simulink model "sim_p_regler_reale_strecke"  (R2016b)
settings: Solver=VariableStepAuto  StartTime=0.0  StopTime=20  FixedStep=1e-3  RelTol=1e3
undefined symbols (not defined in the file or in its folder): param
libraries: simulink x5, simulink_extras x1
settings Model: Creator=nicol  LastModifiedBy=Fritz

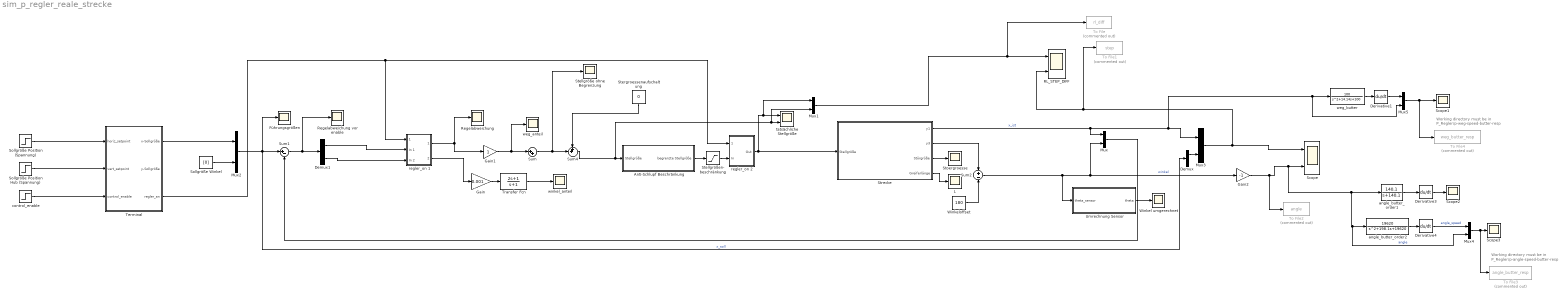
== system sim_p_regler_reale_strecke ==
  note: Working directory must be in
      | P_Regler/p-angle-speed-butter-resp
  note: Working directory must be in
      | P_Regler/p-weg-speed-butter-resp
  Anti-Schlupf Beschränkung : Subsystem
  Demux : Demux  Outputs=2
  Demux1 : Demux  Outputs=2
  Derivative1 : Derivative
  Derivative3 : Derivative
  Derivative4 : Derivative
  Führungsgrößen : Scope
  Gain : Gain  Gain=0.001
  Gain1 : Gain
  Gain2 : Gain  Gain=-1
  L : Scope
  Mux{,1..5} (6 alike) : Mux  Inputs=2
  RL_STEP_DIFF : Scope  NumInputPorts=2
  Regelabweichung : Scope
  Regelabweichung vor enable : Scope
  Scope : Scope  NumInputPorts=2
  Scope1 : Scope
  Scope2 : Scope
  Scope3 : Scope
  Sollgröße Position (Spannung) : Step  SampleTime=0
  Sollgröße Position Hub (Spannung) : Step  Time=2  After=0.5  SampleTime=0
  Sollgröße Winkel : Constant  Value=[0]  VectorParams1D=off
  Stellgröße ohne Begrenzung : Scope
  Stellgrößen- beschränkung : Saturate  UpperLimit=1  LowerLimit=-1
  Stergroessenaufschaltung : Constant  Value=0
  Stoergroesse : Scope
  Strecke : Subsystem
  Sum : Sum  Inputs=|++
  Sum1 : Sum  Inputs=|+-
  Sum2 : Sum  Inputs=+|-
  Sum4 : Sum  Inputs=++|
  Terminal : Subsystem
  To File : ToFile  Commented=on  Filename=rl_diff  SaveFormat=Timeseries
  To File1 : ToFile  Commented=on  Filename=step  SaveFormat=Timeseries
  To File2 : ToFile  Commented=on  Filename=angle  SaveFormat=Timeseries
  To File3 : ToFile  Commented=on  Filename=angle_butter_resp  SaveFormat=Timeseries
  To File4 : ToFile  Commented=on  Filename=weg_butter_resp  SaveFormat=Timeseries
  Transfer Fcn : TransferFcn  Numerator=[2 1]  Denominator=[1 1]
  Umrechnung Sensor : MATLAB Function  TreatAsAtomicUnit=on
  Winkel umgerechnet : Scope
  Winkeloffset : Constant  Value=180
  angle_butter_order1 : TransferFcn  Numerator=[140.1]  Denominator=[1, 140.1]
  angle_butter_order2 : TransferFcn  Numerator=[19620]  Denominator=[1, 198.1, 19620]
  control_enable : Step  Time=0  SampleTime=0
  regler_on 1 : Subsystem
  regler_on 2 : Subsystem
  tatsächliche Stellgröße : Scope  NumInputPorts=2
  weg_anteil : Scope
  weg_butter : TransferFcn  Numerator=[100]  Denominator=[1, 14.14, 100]
  winkel_anteil : Scope
  wires:
  Sum/1 -> Stellgröße ohne Begrenzung/1, Sum4/2
  Sollgröße Winkel/1 -> Mux2/2
  Umrechnung Sensor/1(theta) -> Winkel umgerechnet/1
  Winkeloffset/1 -> Sum2/2
  Sum2/1 -> Umrechnung Sensor/1(theta_sensor), Mux/2, Gain2/1  "winkel"
  Anti-Schlupf Beschränkung/1(begrenzte Stellgröße) -> Stellgrößen- beschränkung/1
  Demux1/1 -> regler_on 1/2(In 1)
  Demux1/2 -> regler_on 1/3(In 2)
  Sum1/1 -> Demux1/1, Regelabweichung vor enable/1
  Mux2/1 -> Demux/1, Sum1/1, Führungsgrößen/1  "x_soll"
  Strecke/1(y1) -> Mux/1, Mux5/2, weg_butter/1, Mux3/1  "x_ist"
  Terminal/3(regler_an) -> regler_on 1/1(regler_ on), regler_on 2/1(regler_ on)
  Strecke/2(y3) -> Sum2/1
  regler_on 1/2(Out 2) -> Gain/1
  regler_on 1/1(Out 1) -> Gain1/1, Regelabweichung/1
  Stellgrößen- beschränkung/1 -> regler_on 2/2(In)
  Sollgröße Position (Spannung)/1 -> Terminal/1(horiz_setpoint)
  control_enable/1 -> Terminal/3(control_enable)
  Sollgröße Position Hub (Spannung)/1 -> Terminal/2(vert_setpoint)
  Terminal/1(x-Sollgröße) -> Mux2/1
  Stergroessenaufschaltung/1 -> Sum4/1
  Strecke/3(Störgröße) -> Stoergroesse/1
  Strecke/4(Greiferlänge) -> L/1
  Mux/1 -> Sum1/2
  Gain/1 -> Transfer Fcn/1
  regler_on 2/1(Out) -> Strecke/1(Stellgröße), Mux1/1, tatsächliche Stellgröße/1
  Sum4/1 -> Mux1/2, tatsächliche Stellgröße/2, Anti-Schlupf Beschränkung/1(Stellgröße)
  Gain1/1 -> weg_anteil/1, Sum/1
  Demux/1 -> Mux3/2
  Mux3/1 -> To File1/1, RL_STEP_DIFF/2, Scope/1
  Mux1/1 -> To File/1, RL_STEP_DIFF/1
  Transfer Fcn/1 -> winkel_anteil/1
  angle_butter_order1/1 -> Derivative3/1
  Derivative3/1 -> Scope2/1
  angle_butter_order2/1 -> Derivative4/1
  Derivative4/1 -> Mux4/1  "angle_speed"
  Gain2/1 -> To File2/1, Mux4/2, angle_butter_order2/1, angle_butter_order1/1, Scope/2  "angle"
  Mux4/1 -> To File3/1, Scope3/1
  weg_butter/1 -> Derivative1/1
  Derivative1/1 -> Mux5/1
  Mux5/1 -> To File4/1, Scope1/1

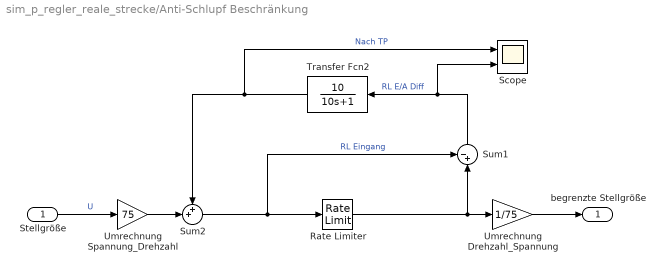
== system sim_p_regler_reale_strecke/Anti-Schlupf Beschränkung ==
  Stellgröße : Inport
  Rate Limiter : RateLimiter  RisingSlewLimit=9.57  FallingSlewLimit=-9.57  SampleTimeMode=inherited
  Scope : Scope  NumInputPorts=2
  Sum1 : Sum  Inputs=-+|
  Sum2 : Sum  Inputs=++|
  Transfer Fcn2 : TransferFcn  Numerator=[10]  Denominator=[10 1]
  Umrechnung Drehzahl_Spannung : Gain  Gain=1/75
  Umrechnung Spannung_Drehzahl : Gain  Gain=75
  begrenzte Stellgröße : Outport
  wires:
  Stellgröße/1 -> Umrechnung Spannung_Drehzahl/1  "U"
  Sum2/1 -> Sum1/1, Rate Limiter/1  "RL Eingang"
  Sum1/1 -> Scope/2, Transfer Fcn2/1  "RL E/A Diff"
  Transfer Fcn2/1 -> Scope/1, Sum2/1  "Nach TP"
  Rate Limiter/1 -> Umrechnung Drehzahl_Spannung/1, Sum1/2
  Umrechnung Spannung_Drehzahl/1 -> Sum2/2
  Umrechnung Drehzahl_Spannung/1 -> begrenzte Stellgröße/1

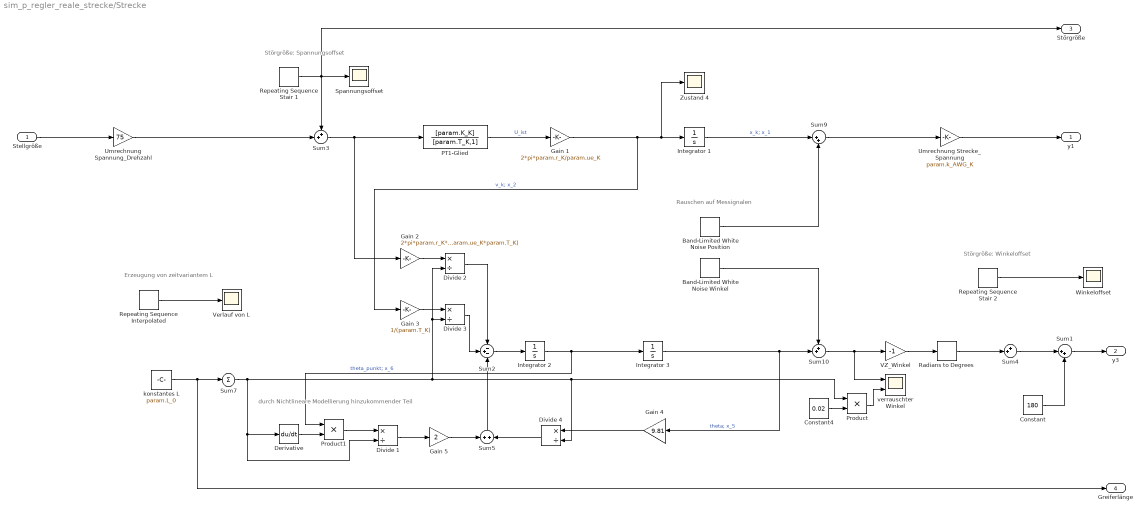
== system sim_p_regler_reale_strecke/Strecke ==
  note: Störgröße: Spannungsoffset
  note: durch Nichtlineare Modellierung hinzukommender Teil
  note: Rauschen auf Messignalen
  note: Erzeugung von zeitvariantem L
  note: Störgröße: Winkeloffset
  Stellgröße : Inport
  Band-Limited White Noise Position : simulink/Sources/Band-Limited White Noise  Cov=[0.0000001]  Ts=0.01  seed=[23341]
  Band-Limited White Noise Winkel : simulink/Sources/Band-Limited White Noise  Cov=[0.000000001]  Ts=0.01  seed=[23341]
  Constant : Constant  Value=180
  Constant4 : Constant  Value=0.02
  Derivative : Derivative
  Divide {1..4} (4 alike) : Product  Inputs=*/
  Gain 1 : Gain  Gain=2*pi*param.r_K/param.ue_K
  Gain 2 : Gain  Gain=2*pi*param.r_K*param.K_K/(param.ue_K*param.T_K)
  Gain 3 : Gain  Gain=1/(param.T_K)
  Gain 4 : Gain  Gain=9.81
  Gain 5 : Gain  Gain=2
  Integrator 1 : Integrator
  Integrator 2 : Integrator
  Integrator 3 : Integrator
  PT1-Glied : TransferFcn  Numerator=[param.K_K]  Denominator=[param.T_K,1]
  Product : Product
  Product1 : Product
  Radians to Degrees : simulink_extras/Transformations/Radians to Degrees
  Repeating Sequence Interpolated : simulink/Sources/Repeating Sequence Interpolated  OutValues=[1.5 1.0 0.7 0.5 0.4 0.3 0.2 0.5 1.5 1.0 0.2 0.2 1.0 1.5 0.5 0.2].'  TimeValues=[0 2 4 6 8 10 12 14 16 18 20 22 24 26 28 30].'  LookUpMeth=Interpolation-Use End Values  tsamp=0.001  OutMin=[]  OutMax=[]  OutDataTypeStr=double  OutputDataTypeScalingMode=double  OutDataType=fixdt(0,8)  OutScaling=2^-10
  Repeating Sequence Stair 1 : simulink/Sources/Repeating Sequence Stair  OutValues=[0.05 0.05 0.05 0.05 0.05].'  tsamp=5  OutMin=[]  OutMax=[]  OutDataTypeStr=double  OutputDataTypeScalingMode=double  OutDataType=fixdt(0,8)  ConRadixGroup=Best Precision: Vector-wise  OutScaling=2^-12
  Repeating Sequence Stair 2 : simulink/Sources/Repeating Sequence Stair  OutValues=[2 2 2 2 2 2].'  tsamp=5  OutMin=[]  OutMax=[]  OutDataTypeStr=double  OutputDataTypeScalingMode=double  OutDataType=fixdt(0,8)  ConRadixGroup=Best Precision: Vector-wise  OutScaling=2^-12
  Spannungsoffset : Scope
  Sum1 : Sum  Inputs=|++
  Sum10 : Sum  Inputs=++|
  Sum2 : Sum  Inputs=-+-
  Sum3 : Sum  Inputs=++|
  Sum4 : Sum  Inputs=++|
  Sum5 : Sum  Inputs=+|+
  Sum7 : Sum  Inputs=|+|
  Sum9 : Sum  Inputs=|++
  Umrechnung Spannung_Drehzahl : Gain  Gain=75
  Umrechnung Strecke_Spannung : Gain  Gain=param.k_AWG_K
  VZ_Winkel : Gain  Gain=-1
  Verlauf von L : Scope
  Winkeloffset : Scope
  Zustand 4 : Scope
  konstantes L : Constant  Value=param.L_0
  verrauschter Winkel : Scope  NumInputPorts=2
  y1 : Outport
  y3 : Outport  Port=2
  Störgröße : Outport  Port=3
  Greiferlänge : Outport  Port=4
  wires:
  PT1-Glied/1 -> Gain 1/1  "U_ist"
  Gain 1/1 -> Zustand 4/1, Integrator 1/1, Gain 3/1  "v_k; x_2"
  Sum2/1 -> Integrator 2/1
  Integrator 2/1 -> Product1/1, Integrator 3/1  "theta_punkt; x_6"
  Sum3/1 -> PT1-Glied/1, Gain 2/1
  Repeating Sequence Stair 1/1 -> Sum3/1, Störgröße/1, Spannungsoffset/1
  Gain 2/1 -> Divide 2/1
  Divide 2/1 -> Sum2/1
  Gain 3/1 -> Divide 3/1
  Divide 3/1 -> Sum2/2
  Gain 4/1 -> Divide 4/1
  Product/1 -> verrauschter Winkel/2
  Constant4/1 -> Product/2
  Integrator 1/1 -> Sum9/1  "x_k; x_1"
  Sum9/1 -> Umrechnung Strecke_Spannung/1
  Divide 4/1 -> Sum5/2
  Sum5/1 -> Sum2/3
  Gain 5/1 -> Sum5/1
  Product1/1 -> Divide 1/1
  Divide 1/1 -> Gain 5/1
  Derivative/1 -> Product1/2
  Stellgröße/1 -> Umrechnung Spannung_Drehzahl/1
  Umrechnung Spannung_Drehzahl/1 -> Sum3/2
  Umrechnung Strecke_Spannung/1 -> y1/1
  Sum10/1 -> VZ_Winkel/1, verrauschter Winkel/1
  Sum1/1 -> y3/1
  Constant/1 -> Sum1/2
  VZ_Winkel/1 -> Radians to Degrees/1
  Band-Limited White Noise Winkel/1 -> Sum10/1
  Integrator 3/1 -> Gain 4/1, Sum10/2  "theta; x_5"
  Sum7/1 -> Divide 1/2, Derivative/1, Divide 3/2, Divide 2/2, Divide 4/2, Product/1
  Sum4/1 -> Sum1/1
  Radians to Degrees/1 -> Sum4/2
  Repeating Sequence Stair 2/1 -> Winkeloffset/1
  Repeating Sequence Interpolated/1 -> Verlauf von L/1
  konstantes L/1 -> Greiferlänge/1, Sum7/1
  Band-Limited White Noise Position/1 -> Sum9/2

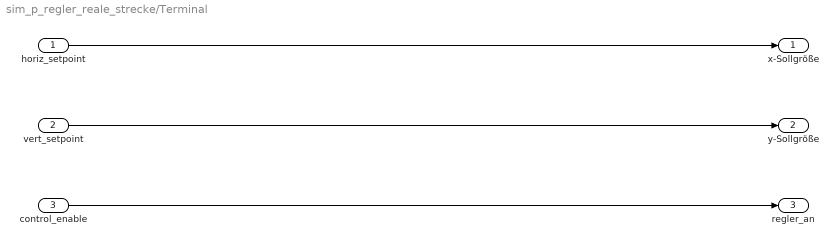
== system sim_p_regler_reale_strecke/Terminal ==
  horiz_setpoint : Inport
  vert_setpoint : Inport  Port=2
  control_enable : Inport  Port=3
  x-Sollgröße : Outport
  y-Sollgröße : Outport  Port=2
  regler_an : Outport  Port=3
  wires:
  horiz_setpoint/1 -> x-Sollgröße/1
  vert_setpoint/1 -> y-Sollgröße/1
  control_enable/1 -> regler_an/1

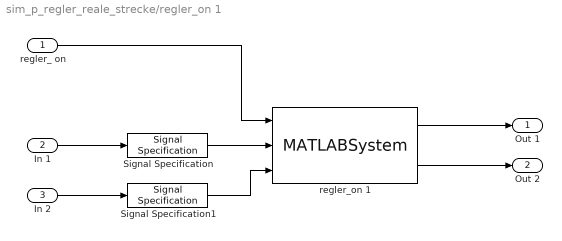
== system sim_p_regler_reale_strecke/regler_on 1 ==
  regler_ on : Inport
  In 1 : Inport  Port=2
  In 2 : Inport  Port=3
  Signal Specification : SignalSpecification  Dimensions=1
  Signal Specification1 : SignalSpecification  Dimensions=1
  regler_on 1 : MATLABSystem  System=regler_switch_2  SimulateUsing=Code generation
      mask Type: regler_switch_2
      mask Display:
      | disp('regler_switch_2');
      | port_label('input',1,'regler_on');
      | port_label('input',2,'input1');
      | port_label('input',3,'input2');
      | port_label('output',1,'y1');
      | port_label('output',2,'y2');
  Out 1 : Outport
  Out 2 : Outport  Port=2
  wires:
  regler_on 1/1 -> Out 1/1
  regler_on 1/2 -> Out 2/1
  In 2/1 -> Signal Specification1/1
  In 1/1 -> Signal Specification/1
  Signal Specification/1 -> regler_on 1/2
  Signal Specification1/1 -> regler_on 1/3
  regler_ on/1 -> regler_on 1/1

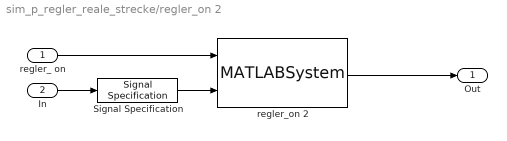
== system sim_p_regler_reale_strecke/regler_on 2 ==
  regler_ on : Inport
  In : Inport  Port=2
  Signal Specification : SignalSpecification  Dimensions=1
  regler_on 2 : MATLABSystem  System=regler_switch_1  SimulateUsing=Code generation
      mask Type: regler_switch_1
      mask Display:
      | disp('regler_switch_1');
      | port_label('input',1,'regler_on');
      | port_label('input',2,'input');
      | port_label('output',1,'y');
  Out : Outport
  wires:
  regler_ on/1 -> regler_on 2/1
  regler_on 2/1 -> Out/1
  Signal Specification/1 -> regler_on 2/2
  In/1 -> Signal Specification/1

== matlab function sim_p_regler_reale_strecke/Umrechnung Sensor ==
  data: theta_sensor input; theta output
function theta  = sensorWinkel(theta_sensor)
% berechnet aus dem gemessenen Winkel den tatsächlichen Winkel des
% Lasthebers

% l_verb: Länge des Verbindungsstücks
% l_welle: Abstand der beiden Wellen

% Parameter für die Winkelumrechnung
l_verb = 0.109; % m %
l_welle = 0.0575; % m %

theta = asin(sin(theta_sensor) * (l_verb / sqrt(l_welle^2 + l_verb^2 - (2 * l_verb * l_welle * cos(theta_sensor)))));
